simulink model "kalman_ac_sim"  (R2025b)
settings: Solver=VariableStepAuto  StartTime=0.0  StopTime=StopTime  RelTol=1e-3
values from neighbouring files (symbols this model uses):
  B = single([0.5*dt^2 0; 0 0.5*dt^2; dt 0; 0 dt])    [model_test.m]
  C = eye(4) / (H*H' + R)    [model_test.m]
  dt = 0.02    [model_test.m]
  F = single([1 0 dt 0; 0 1 0 dt; 0 0 1 0; 0 0 0 1])    [model_test.m]
  H = single(diag([1,1,1,1]))    [model_test.m]
  Q = single(0.1 * eye(4))    [model_test.m]
  time = single(0:dt:StopTime)    [model_test.m]
undefined symbols (not defined in the file or in its folder): T1, T10, T11, T12, T13, T14, T15, T16, T2, T3, T4, T5, T6, T7, T8, T9
libraries: dspsrcs4 x3, hdlsllib x2
settings Model: Creator=stefa  LastModifiedBy=david
settings OptimizationCC: BlockReduction=off  ConditionallyExecuteInputs=off

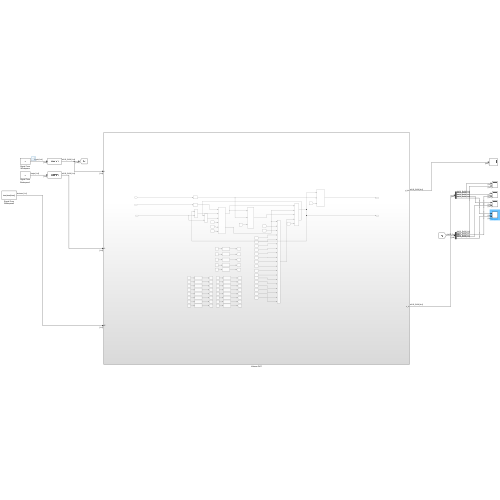
[thumbnail: Simulink's stored preview of the top-level diagram]
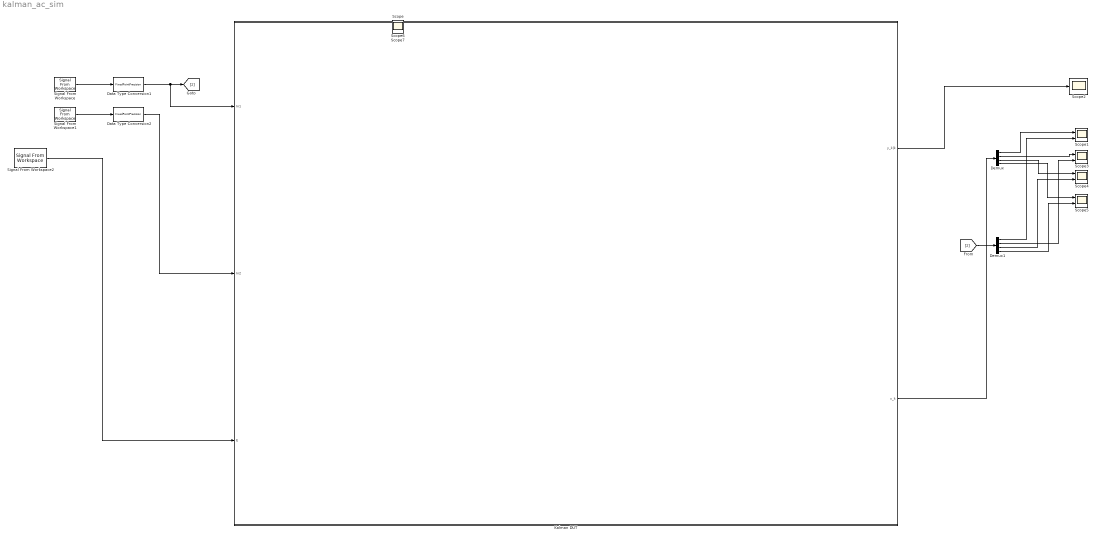
== system kalman_ac_sim ==
  Data Type Conversion1 : DataTypeConversion  OutDataTypeStr=FixedPointPrecision  SaturateOnIntegerOverflow=off  RndMeth=Floor
  Data Type Conversion2 : DataTypeConversion  OutDataTypeStr=FixedPointPrecision  SaturateOnIntegerOverflow=off  RndMeth=Floor
  Demux : Demux
  Demux1 : Demux
  Kalman DUT : Subsystem
  Scope{1,3..5} (4 alike) : Scope  NumInputPorts=2
      Scope1 settings: ActiveDisplayYMinimum=-0.51561176776885986  ActiveDisplayYMaximum=2.7327185869216919  DataLoggingSaveFormat=Array
      Scope3 settings: ActiveDisplayYMinimum=-0.48612570762634272  ActiveDisplayYMaximum=2.5642850399017334  DataLoggingVariableName=ScopeData2  DataLoggingSaveFormat=Array
      Scope4 settings: ActiveDisplayYMinimum=-1.6568914651870728  ActiveDisplayYMaximum=1.5055176019668579  DataLoggingVariableName=ScopeData3  DataLoggingSaveFormat=Array
      Scope5 settings: ActiveDisplayYMinimum=-1.4646996259689331  ActiveDisplayYMaximum=1.4755533933639526  DataLoggingVariableName=ScopeData4  DataLoggingSaveFormat=Array
  Scope{,2,6..7} (4 alike) : Scope
      Scope2 settings: ActiveDisplayYMinimum=-0.011525178669385456  ActiveDisplayYMaximum=0.00587966952456793  DataLoggingSaveFormat=Array
      Scope settings: ActiveDisplayYMinimum=-9.1353842219735029  ActiveDisplayYMaximum=57.624373102579447  DataLoggingVariableName=ScopeData5
      Scope6 settings: ActiveDisplayYMinimum=-1  ActiveDisplayYMaximum=1  DataLoggingVariableName=ScopeData6
      Scope7 settings: ActiveDisplayYMinimum=-0.035523056983947747  ActiveDisplayYMaximum=0.31970751285552979  DataLoggingVariableName=ScopeData7
  Signal From Workspace : dspsrcs4/Signal From Workspace  X=z  Ts=dt  nsamps=1  OutputAfterFinalValue=Setting to zero  ignoreOrWarnInputAndFrameLengths=off  OutputFrames=off
  Signal From Workspace1 : dspsrcs4/Signal From Workspace  X=u  Ts=dt  nsamps=1  OutputAfterFinalValue=Setting to zero  ignoreOrWarnInputAndFrameLengths=off  OutputFrames=off
  Signal From Workspace2 : dspsrcs4/Signal From Workspace  X=true(size(time))  Ts=dt  nsamps=1  OutputAfterFinalValue=Setting to zero  ignoreOrWarnInputAndFrameLengths=off  OutputFrames=off
  wires:
  Demux/1 -> Scope1/1
  Demux/2 -> Scope3/1
  Demux/3 -> Scope4/1
  Demux/4 -> Scope5/1
  [z] -> Demux1/1
  Demux1/1 -> Scope1/2
  Demux1/2 -> Scope3/2
  Demux1/3 -> Scope4/2
  Demux1/4 -> Scope5/2
  Signal From Workspace/1 -> Data Type Conversion1/1
  Signal From Workspace1/1 -> Data Type Conversion2/1
  Kalman DUT/1(y_k|k) -> Scope2/1
  Kalman DUT/2(x_k) -> Demux/1
  Data Type Conversion1/1 -> Kalman DUT/1(In1), [z]
  Data Type Conversion2/1 -> Kalman DUT/2(In2)
  Signal From Workspace2/1 -> Kalman DUT/3(E)

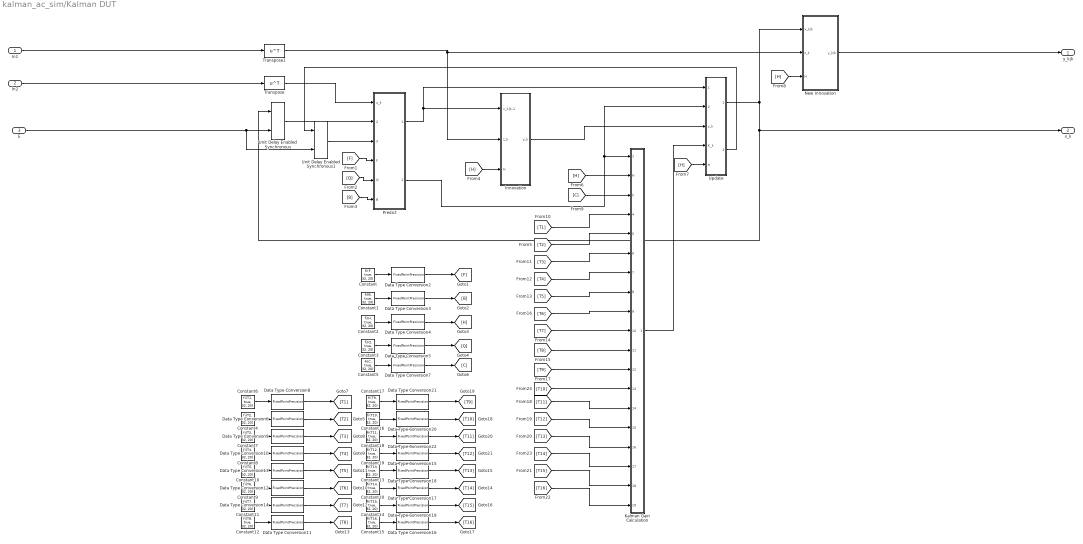
== system kalman_ac_sim/Kalman DUT ==
  In1 : Inport
  In2 : Inport  Port=2
  E : Inport  Port=3
  Constant : Constant  Value=fi(F, true, 32, 20)
  Constant1 : Constant  Value=fi(B, true, 32, 20)
  Constant10 : Constant  Value=fi(T5, true, 32, 20)
  Constant11 : Constant  Value=fi(T7, true, 32, 20)
  Constant12 : Constant  Value=fi(T8, true, 32, 20)
  Constant13 : Constant  Value=fi(T13, true, 32, 20)
  Constant14 : Constant  Value=fi(T15, true, 32, 20)
  Constant15 : Constant  Value=fi(T16, true, 32, 20)
  Constant16 : Constant  Value=fi(T10, true, 32, 20)
  Constant17 : Constant  Value=fi(T9, true, 32, 20)
  Constant18 : Constant  Value=fi(T11, true, 32, 20)
  Constant19 : Constant  Value=fi(T12, true, 32, 20)
  Constant2 : Constant  Value=fi(H, true, 32, 20)
  Constant20 : Constant  Value=fi(T14, true, 32, 20)
  Constant3 : Constant  Value=fi(Q, true, 32, 20)
  Constant4 : Constant  Value=fi(T2, true, 32, 20)
  Constant5 : Constant  Value=fi(C, true, 32, 20)
  Constant6 : Constant  Value=fi(T1, true, 32, 20)
  Constant7 : Constant  Value=fi(T3, true, 32, 20)
  Constant8 : Constant  Value=fi(T4, true, 32, 20)
  Constant9 : Constant  Value=fi(T6, true, 32, 20)
  Data Type Conversion{2..22} (21 alike) : DataTypeConversion  OutDataTypeStr=FixedPointPrecision  SaturateOnIntegerOverflow=off  RndMeth=Floor
  Innovation : Subsystem
  Kalman Gain Calculation : Subsystem
  New Innovation : Subsystem
  Predict : Subsystem
  Transpose : Math  Operator=transpose  SignedPower=on  RndMeth=Zero
  Transpose1 : Math  Operator=transpose  SignedPower=on  RndMeth=Zero
  Unit Delay Enabled Synchronous : hdlsllib/Discrete/Unit Delay Enabled Synchronous  InitialCondition=0.0  SampleTime=-1
  Unit Delay Enabled Synchronous1 : hdlsllib/Discrete/Unit Delay Enabled Synchronous  InitialCondition=0.0  SampleTime=-1
  Update : Subsystem
  y_k|k : Outport
  x_k : Outport  Port=2
  wires:
  Constant17/1 -> Data Type Conversion21/1
  Kalman Gain Calculation/1(K_k) -> Update/4(K_k)
  [T15] -> Kalman Gain Calculation/18(T15)
  Constant3/1 -> Data Type Conversion5/1
  Data Type Conversion10/1 -> [T4]
  [H] -> Update/5(H)
  Data Type Conversion7/1 -> [C]
  Constant19/1 -> Data Type Conversion15/1
  Constant4/1 -> Data Type Conversion6/1
  Constant13/1 -> Data Type Conversion18/1
  Unit Delay Enabled Synchronous/1 -> Predict/2(x_k-1|k-1)
  Predict/2(P_k|k-1) -> Update/2(P_k|k-1), Kalman Gain Calculation/1(P_k|k-1)
  Constant8/1 -> Data Type Conversion10/1
  Data Type Conversion16/1 -> [T16]
  [T1] -> Kalman Gain Calculation/4(T1)
  Constant2/1 -> Data Type Conversion4/1
  [C] -> Kalman Gain Calculation/3(C)
  [H] -> Kalman Gain Calculation/2(H)
  Data Type Conversion9/1 -> [T3]
  E/1 -> Unit Delay Enabled Synchronous/2, Unit Delay Enabled Synchronous1/2
  Transpose1/1 -> Innovation/2(z_k), New Innovation/2(z_k)
  Data Type Conversion15/1 -> [T12]
  Predict/1(x_k|k-1) -> Update/1(x_k|k-1), Innovation/1(x_k|k-1)
  Data Type Conversion18/1 -> [T13]
  Constant5/1 -> Data Type Conversion7/1
  Constant/1 -> Data Type Conversion2/1
  Constant10/1 -> Data Type Conversion13/1
  Data Type Conversion3/1 -> [B]
  [T6] -> Kalman Gain Calculation/9(T6)
  Constant18/1 -> Data Type Conversion22/1
  [H] -> Innovation/3(H)
  Constant12/1 -> Data Type Conversion11/1
  Data Type Conversion8/1 -> [T1]
  Transpose/1 -> Predict/1(u_k)
  Data Type Conversion4/1 -> [H]
  Innovation/1(y_k) -> Update/3(y_k)
  Constant7/1 -> Data Type Conversion9/1
  [Q] -> Predict/5(Q)
  Data Type Conversion17/1 -> [T14]
  Update/2(P_k|k) -> Unit Delay Enabled Synchronous1/1
  Unit Delay Enabled Synchronous1/1 -> Predict/3(P_k-1|k-1)
  Data Type Conversion5/1 -> [Q]
  Data Type Conversion2/1 -> [F]
  [H] -> New Innovation/3(H)
  Data Type Conversion6/1 -> [T2]
  Constant16/1 -> Data Type Conversion20/1
  Data Type Conversion19/1 -> [T15]
  Update/1(x_k|k) -> New Innovation/1(x_k|k), Unit Delay Enabled Synchronous/1, x_k/1
  [T10] -> Kalman Gain Calculation/13(T10)
  Constant6/1 -> Data Type Conversion8/1
  Constant1/1 -> Data Type Conversion3/1
  [B] -> Predict/6(B)
  [F] -> Predict/4(F)
  Constant15/1 -> Data Type Conversion16/1
  Constant20/1 -> Data Type Conversion17/1
  Data Type Conversion21/1 -> [T9]
  [T12] -> Kalman Gain Calculation/15(T12)
  [T9] -> Kalman Gain Calculation/12(T9)
  Data Type Conversion11/1 -> [T8]
  Constant14/1 -> Data Type Conversion19/1
  Data Type Conversion22/1 -> [T11]
  Data Type Conversion20/1 -> [T10]
  Data Type Conversion13/1 -> [T5]
  Data Type Conversion12/1 -> [T6]
  Constant11/1 -> Data Type Conversion14/1
  Data Type Conversion14/1 -> [T7]
  Constant9/1 -> Data Type Conversion12/1
  [T11] -> Kalman Gain Calculation/14(T11)
  [T16] -> Kalman Gain Calculation/19(T16)
  [T13] -> Kalman Gain Calculation/16(T13)
  [T7] -> Kalman Gain Calculation/10(T7)
  [T8] -> Kalman Gain Calculation/11(T8)
  [T3] -> Kalman Gain Calculation/6(T3)
  [T2] -> Kalman Gain Calculation/5(T2)
  [T5] -> Kalman Gain Calculation/8(T5)
  [T4] -> Kalman Gain Calculation/7(T4)
  [T14] -> Kalman Gain Calculation/17(T14)
  In2/1 -> Transpose/1
  New Innovation/1(y_k|k) -> y_k|k/1
  In1/1 -> Transpose1/1

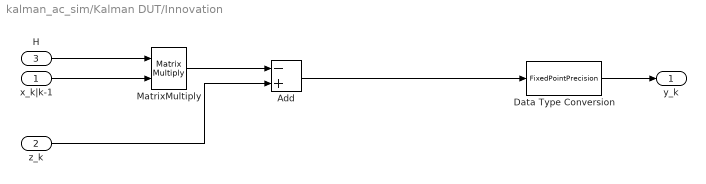
== system kalman_ac_sim/Kalman DUT/Innovation ==
  x_k|k-1 : Inport
  z_k : Inport  Port=2
  H : Inport  Port=3
  Add : Sum  Inputs=-+
  Data Type Conversion : DataTypeConversion  OutDataTypeStr=FixedPointPrecision  SaturateOnIntegerOverflow=off  RndMeth=Floor
  MatrixMultiply : Product  Multiplication=Matrix(*)
  y_k : Outport
  wires:
  x_k|k-1/1 -> MatrixMultiply/2
  MatrixMultiply/1 -> Add/1
  z_k/1 -> Add/2
  Add/1 -> Data Type Conversion/1
  H/1 -> MatrixMultiply/1
  Data Type Conversion/1 -> y_k/1

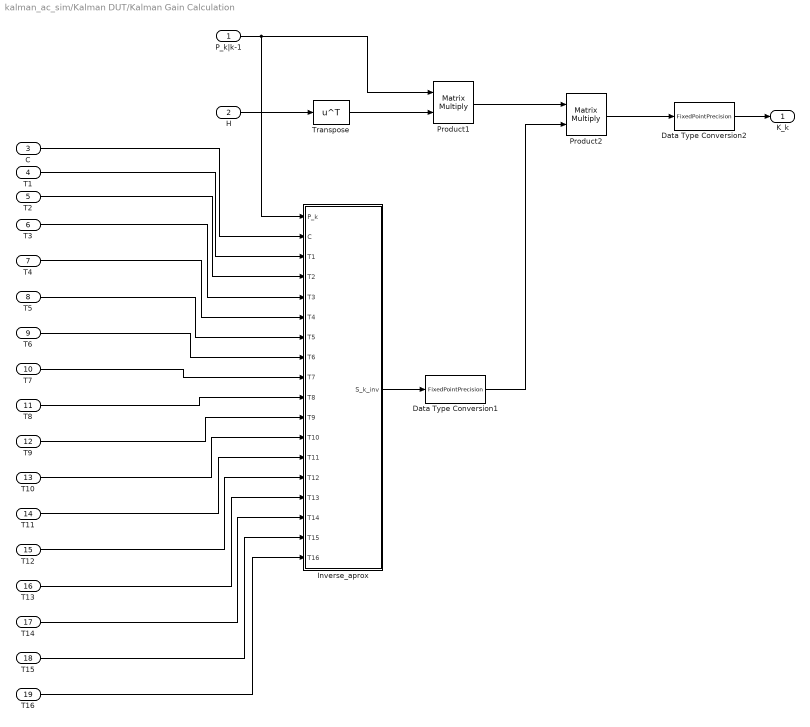
== system kalman_ac_sim/Kalman DUT/Kalman Gain Calculation ==
  P_k|k-1 : Inport
  H : Inport  Port=2
  C : Inport  Port=3
  T1 : Inport  Port=4
  T2 : Inport  Port=5
  T3 : Inport  Port=6
  T4 : Inport  Port=7
  T5 : Inport  Port=8
  T6 : Inport  Port=9
  T7 : Inport  Port=10
  T8 : Inport  Port=11
  T9 : Inport  Port=12
  T10 : Inport  Port=13
  T11 : Inport  Port=14
  T12 : Inport  Port=15
  T13 : Inport  Port=16
  T14 : Inport  Port=17
  T15 : Inport  Port=18
  T16 : Inport  Port=19
  Data Type Conversion1 : DataTypeConversion  OutDataTypeStr=FixedPointPrecision  SaturateOnIntegerOverflow=off  RndMeth=Floor
  Data Type Conversion2 : DataTypeConversion  OutDataTypeStr=FixedPointPrecision  SaturateOnIntegerOverflow=off  RndMeth=Floor
  Inverse_aprox : MATLAB Function  TreatAsAtomicUnit=on
  Product1 : Product  Multiplication=Matrix(*)
  Product2 : Product  Multiplication=Matrix(*)
  Transpose : Math  Operator=transpose  SignedPower=on  RndMeth=Zero
  K_k : Outport
  wires:
  H/1 -> Transpose/1
  P_k|k-1/1 -> Product1/1, Inverse_aprox/1(P_k)
  Transpose/1 -> Product1/2
  Inverse_aprox/1(S_k_inv) -> Data Type Conversion1/1
  Product2/1 -> Data Type Conversion2/1
  Product1/1 -> Product2/1
  Data Type Conversion1/1 -> Product2/2
  Data Type Conversion2/1 -> K_k/1
  C/1 -> Inverse_aprox/2(C)
  T1/1 -> Inverse_aprox/3(T1)
  T2/1 -> Inverse_aprox/4(T2)
  T3/1 -> Inverse_aprox/5(T3)
  T4/1 -> Inverse_aprox/6(T4)
  T5/1 -> Inverse_aprox/7(T5)
  T6/1 -> Inverse_aprox/8(T6)
  T7/1 -> Inverse_aprox/9(T7)
  T8/1 -> Inverse_aprox/10(T8)
  T9/1 -> Inverse_aprox/11(T9)
  T10/1 -> Inverse_aprox/12(T10)
  T11/1 -> Inverse_aprox/13(T11)
  T12/1 -> Inverse_aprox/14(T12)
  T13/1 -> Inverse_aprox/15(T13)
  T14/1 -> Inverse_aprox/16(T14)
  T15/1 -> Inverse_aprox/17(T15)
  T16/1 -> Inverse_aprox/18(T16)

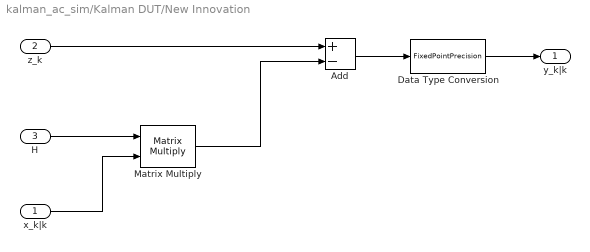
== system kalman_ac_sim/Kalman DUT/New Innovation ==
  x_k|k : Inport
  z_k : Inport  Port=2
  H : Inport  Port=3
  Add : Sum  Inputs=+-
  Data Type Conversion : DataTypeConversion  OutDataTypeStr=FixedPointPrecision  SaturateOnIntegerOverflow=off  RndMeth=Floor
  Matrix Multiply : Product  Multiplication=Matrix(*)
  y_k|k : Outport
  wires:
  z_k/1 -> Add/1
  H/1 -> Matrix Multiply/1
  x_k|k/1 -> Matrix Multiply/2
  Matrix Multiply/1 -> Add/2
  Add/1 -> Data Type Conversion/1
  Data Type Conversion/1 -> y_k|k/1

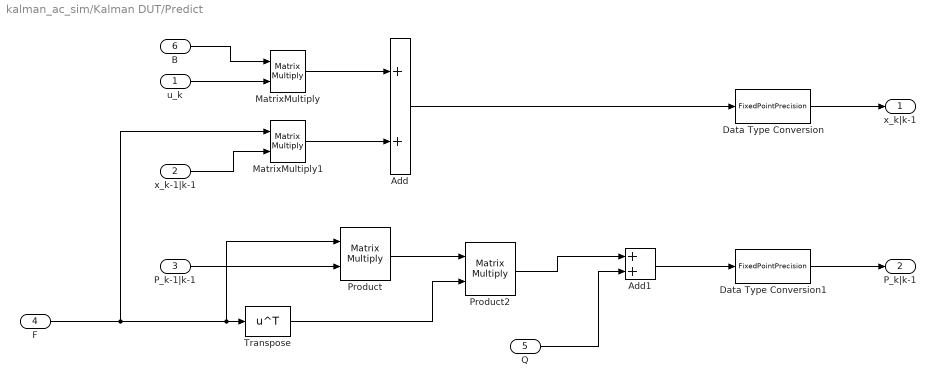
== system kalman_ac_sim/Kalman DUT/Predict ==
  u_k : Inport
  x_k-1|k-1 : Inport  Port=2
  P_k-1|k-1 : Inport  Port=3
  F : Inport  Port=4
  Q : Inport  Port=5
  B : Inport  Port=6
  Add : Sum
  Add1 : Sum
  Data Type Conversion : DataTypeConversion  OutDataTypeStr=FixedPointPrecision  SaturateOnIntegerOverflow=off  RndMeth=Floor
  Data Type Conversion1 : DataTypeConversion  OutDataTypeStr=FixedPointPrecision  SaturateOnIntegerOverflow=off  RndMeth=Floor
  MatrixMultiply : Product  Multiplication=Matrix(*)
  MatrixMultiply1 : Product  Multiplication=Matrix(*)
  Product : Product  Multiplication=Matrix(*)
  Product2 : Product  Multiplication=Matrix(*)
  Transpose : Math  Operator=transpose  SignedPower=on  RndMeth=Zero
  x_k|k-1 : Outport
  P_k|k-1 : Outport  Port=2
  wires:
  x_k-1|k-1/1 -> MatrixMultiply1/2
  Add/1 -> Data Type Conversion/1
  MatrixMultiply1/1 -> Add/2
  MatrixMultiply/1 -> Add/1
  P_k-1|k-1/1 -> Product/2
  Q/1 -> Add1/2
  Add1/1 -> Data Type Conversion1/1
  Product2/1 -> Add1/1
  Product/1 -> Product2/1
  Transpose/1 -> Product2/2
  B/1 -> MatrixMultiply/1
  F/1 -> MatrixMultiply1/1, Transpose/1, Product/1
  Data Type Conversion/1 -> x_k|k-1/1
  Data Type Conversion1/1 -> P_k|k-1/1
  u_k/1 -> MatrixMultiply/2

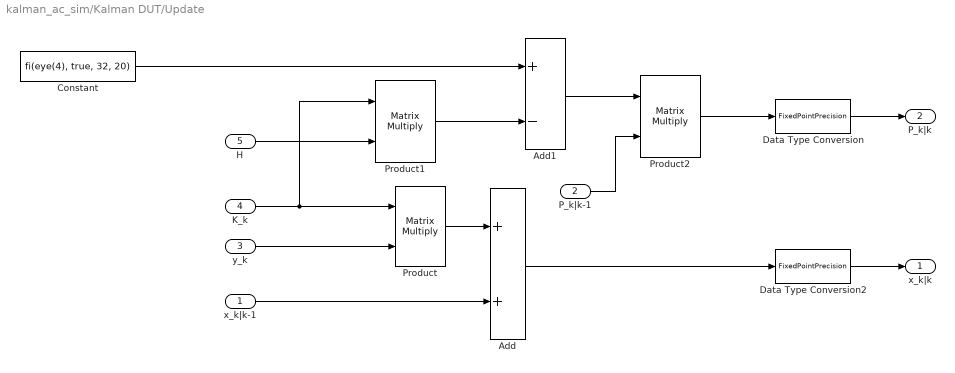
== system kalman_ac_sim/Kalman DUT/Update ==
  x_k|k-1 : Inport
  P_k|k-1 : Inport  Port=2
  y_k : Inport  Port=3
  K_k : Inport  Port=4
  H : Inport  Port=5
  Add : Sum
  Add1 : Sum  Inputs=+-
  Constant : Constant  Value=fi(eye(4), true, 32, 20)
  Data Type Conversion : DataTypeConversion  OutDataTypeStr=FixedPointPrecision  SaturateOnIntegerOverflow=off  RndMeth=Floor
  Data Type Conversion2 : DataTypeConversion  OutDataTypeStr=FixedPointPrecision  SaturateOnIntegerOverflow=off  RndMeth=Floor
  Product : Product  Multiplication=Matrix(*)
  Product1 : Product  Multiplication=Matrix(*)
  Product2 : Product  Multiplication=Matrix(*)
  x_k|k : Outport
  P_k|k : Outport  Port=2
  wires:
  K_k/1 -> Product1/1, Product/1
  y_k/1 -> Product/2
  Product/1 -> Add/1
  x_k|k-1/1 -> Add/2
  Add/1 -> Data Type Conversion2/1
  H/1 -> Product1/2
  Product1/1 -> Add1/2
  P_k|k-1/1 -> Product2/2
  Add1/1 -> Product2/1
  Product2/1 -> Data Type Conversion/1
  Constant/1 -> Add1/1
  Data Type Conversion/1 -> P_k|k/1
  Data Type Conversion2/1 -> x_k|k/1

== matlab function kalman_ac_sim/Kalman DUT/Kalman Gain Calculation/Inverse_aprox ==
  data: S_k_inv output; P_k input; C input; T1 input; T2 input; T3 input; T4 input; T5 input; T6 input; T7 input; T8 input; T9 input; T10 input; T11 input; T12 input; T13 input; T14 input; T15 input; T16 input
function S_k_inv = inverse_aprox(P_k, C, T1, T2, T3, T4, T5, T6, T7, T8, T9, T10, T11, T12, T13, T14, T15, T16)
    Z = P_k - fi(eye(4),true, 66, 40);
    sum = fi(zeros(4,4),true, 66, 40);
    sum = sum + T1*Z(1,1);
    sum = sum + T2*Z(1,2);
    sum = sum + T3*Z(1,3);
    sum = sum + T4*Z(1,4);
    sum = sum + T5*Z(2,1);
    sum = sum + T6*Z(2,2);
    sum = sum + T7*Z(2,3);
    sum = sum + T8*Z(2,4);
    sum = sum + T9*Z(3,1);
    sum = sum + T10*Z(3,2);
    sum = sum + T11*Z(3,3);
    sum = sum + T12*Z(3,4);
    sum = sum + T13*Z(4,1);
    sum = sum + T14*Z(4,2);
    sum = sum + T15*Z(4,3);
    sum = sum + T16*Z(4,4);    
    S_k_inv = C - fi(sum, true, 32, 20);
end
